simulink model "drone_nonlinear_full_compare"  (R2018a)
settings: Solver=VariableStepAuto  StartTime=0.0  StopTime=20  RelTol=1e-3
undefined symbols (not defined in the file): c, est_c_A, est_c_B, est_c_C, est_c_D, g, Ix, Iy, Iz, l, m, q, rpm, simulation_sampling_ts
libraries: simulink x8
settings Model: Creator=ros  LastModifiedBy=ros

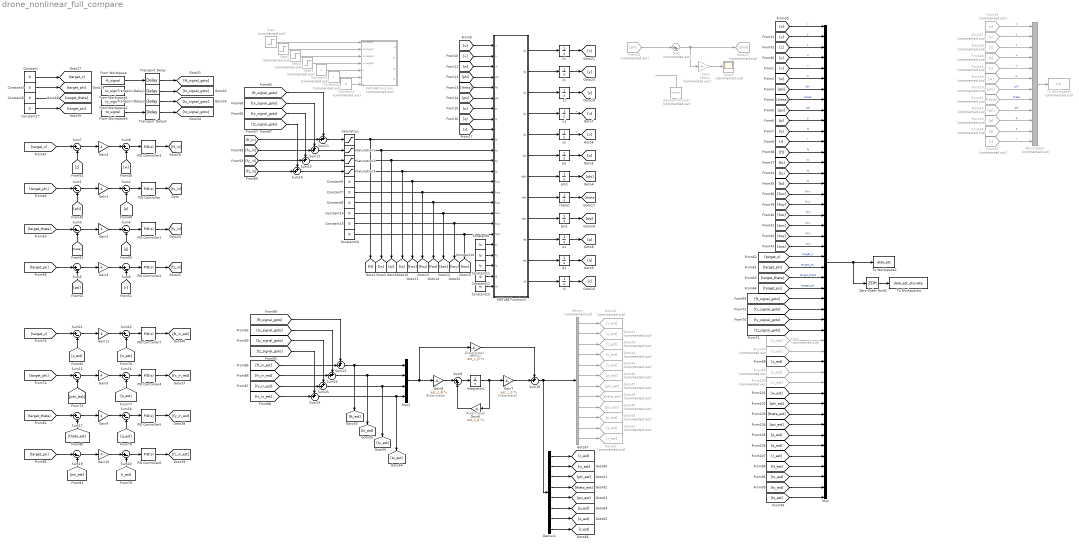
== system drone_nonlinear_full_compare ==
  note: B(estimate)
  note: C(estimate)
  note: A(estimate)
  note: D(estimate)
  Bus Creator : BusCreator  Commented=on  Inputs=12
  Constant{,3,5..8,14..17} (10 alike) : Constant  Value=0
  Constant1 : Constant  Commented=on  Value=l
  Constant10 : Constant  Value=Iy
  Constant11 : Constant  Value=Iz
  Constant12 : Constant  Value=g
  Constant13 : Constant  Value=m
  Constant2 : Constant  Commented=on  Value=c
  Constant4 : Constant  Commented=on  Value=q
  Constant9 : Constant  Value=Ix
  Demux : Demux  Commented=on  Outputs=12
  Demux1 : Demux  Outputs=8
  From : From  Commented=on  GotoTag=x_est
  From Workspace : FromWorkspace  VariableName=ft_signal  SampleTime=0
  From Workspace1 : FromWorkspace  VariableName=tx_signal  SampleTime=0
  From Workspace2 : FromWorkspace  VariableName=ty_signal  SampleTime=0
  From Workspace3 : FromWorkspace  VariableName=tz_signal  SampleTime=0
  From100 : From  Commented=on  GotoTag=v_est
  From18 : From  Commented=on  GotoTag=v
  From19 : From  Commented=on  GotoTag=w
  From20 : From  Commented=on  GotoTag=phi
  From21 : From  Commented=on  GotoTag=theta
  From22 : From  Commented=on  GotoTag=psi
  From23 : From  Commented=on  GotoTag=p
  From24 : From  Commented=on  GotoTag=q
  From25 : From  Commented=on  GotoTag=r
  From26 : From  Commented=on  GotoTag=u
  From27 : From  Commented=on  GotoTag=y
  From28 : From  Commented=on  GotoTag=z
  From29 : From  Commented=on  GotoTag=x
  From44 : From  Commented=on  GotoTag=phi
  From97 : From  Commented=on  GotoTag=y_est
  From99 : From  Commented=on  GotoTag=u_est
  Gain : Gain  Commented=on  Gain=180/pi
  Gain{1..5,9..11} (8 alike) : Gain  Gain=4
  Gain12 : Gain  Gain=est_c_D  Multiplication=Matrix(K*u)
  Gain6 : Gain  Gain=est_c_A  Multiplication=Matrix(K*u)
  Gain7 : Gain  Gain=est_c_C  Multiplication=Matrix(K*u)
  Gain8 : Gain  Gain=est_c_B  Multiplication=Matrix(K*u)
  Goto23 : Goto  Commented=on  GotoTag=phid
  Goto41 : Goto  Commented=on  GotoTag=x_est
  Goto42 : Goto  Commented=on  GotoTag=y_est
  Goto43 : Goto  Commented=on  GotoTag=z_est
  Goto44 : Goto  Commented=on  GotoTag=u_est
  Goto45 : Goto  Commented=on  GotoTag=v_est
  Goto46 : Goto  Commented=on  GotoTag=w_est
  Goto47 : Goto  Commented=on  GotoTag=phi_est
  Goto48 : Goto  Commented=on  GotoTag=theta_est
  Goto49 : Goto  Commented=on  GotoTag=psi_est
  Goto50 : Goto  Commented=on  GotoTag=p_est
  Goto51 : Goto  Commented=on  GotoTag=q_est
  Goto52 : Goto  Commented=on  GotoTag=r_est
  Integrator1 : Integrator
  MATLAB Function : MATLAB Function  Commented=on  TreatAsAtomicUnit=on
  MATLAB Function2 : MATLAB Function  TreatAsAtomicUnit=on
  Mux : Mux  Inputs=46
  Mux1 : Mux
  PID Controller{,1..2,4..6} (6 alike) : simulink/Continuous/PID Controller  Controller=PID  TimeDomain=Continuous-time  SampleTime=-1  IntegratorMethod=Forward Euler  FilterMethod=Forward Euler  Form=Parallel  UseFilter=on  ControllerParametersSource=internal  P=1.5  I=1.5  D=0  N=100  InitialConditionSource=internal  InitialConditionForIntegrator=0  InitialConditionForFilter=0  ExternalReset=none  LimitOutput=off  UpperSaturationLimit=inf  LowerSaturationLimit=-inf  LinearizeAsGain=on  AntiWindupMode=none  Kb=1  TrackingMode=off  Kt=1  PParamMin=[]  PParamMax=[]  IParamMin=[]  IParamMax=[]  DParamMin=[]  DParamMax=[]  NParamMin=[]  NParamMax=[]  KbParamMin=[]  KbParamMax=[]  KtParamMin=[]  KtParamMax=[]  POutMin=[]  POutMax=[]  IOutMin=[]  IOutMax=[]  DOutMin=[]  DOutMax=[]  NOutMin=[]  NOutMax=[]  KbOutMin=[]  KbOutMax=[]  KtOutMin=[]  KtOutMax=[]  IntegratorOutMin=[]  IntegratorOutMax=[]  FilterOutMin=[]  FilterOutMax=[]  SumOutMin=[]  SumOutMax=[]  SumI1OutMin=[]  SumI1OutMax=[]  SumI2OutMin=[]  SumI2OutMax=[]  SumI3OutMin=[]  SumI3OutMax=[]  SumDOutMin=[]  SumDOutMax=[]  SaturationOutMin=[]  SaturationOutMax=[]  IntegratorContinuousStateAttributes=''  IntegratorStateMustResolveToSignalObject=off  IntegratorRTWStateStorageClass=Auto  FilterContinuousStateAttributes=''  FilterStateMustResolveToSignalObject=off  FilterRTWStateStorageClass=Auto  DifferentiatorICPrevScaledInput=0  DifferentiatorOutMin=[]  DifferentiatorOutMax=[]  FilterDiffOutCoefMin=[]  FilterDiffOutCoefMax=[]  SumDenOutMin=[]  SumDenOutMax=[]  SumNumOutMin=[]  SumNumOutMax=[]  ReciprocalOutMin=[]  ReciprocalOutMax=[]  DivideOutMin=[]  DivideOutMax=[]  TunerSelectOption=Transfer Function Based (PID Tuner App)
  PID Controller3 : simulink/Continuous/PID Controller  Controller=PID  TimeDomain=Continuous-time  SampleTime=-1  IntegratorMethod=Forward Euler  FilterMethod=Forward Euler  Form=Parallel  UseFilter=on  ControllerParametersSource=internal  P=7  I=6  D=0.7  N=100  InitialConditionSource=internal  InitialConditionForIntegrator=0  InitialConditionForFilter=0  ExternalReset=none  LimitOutput=off  UpperSaturationLimit=inf  LowerSaturationLimit=-inf  LinearizeAsGain=on  AntiWindupMode=none  Kb=1  TrackingMode=off  Kt=1  PParamMin=[]  PParamMax=[]  IParamMin=[]  IParamMax=[]  DParamMin=[]  DParamMax=[]  NParamMin=[]  NParamMax=[]  KbParamMin=[]  KbParamMax=[]  KtParamMin=[]  KtParamMax=[]  POutMin=[]  POutMax=[]  IOutMin=[]  IOutMax=[]  DOutMin=[]  DOutMax=[]  NOutMin=[]  NOutMax=[]  KbOutMin=[]  KbOutMax=[]  KtOutMin=[]  KtOutMax=[]  IntegratorOutMin=[]  IntegratorOutMax=[]  FilterOutMin=[]  FilterOutMax=[]  SumOutMin=[]  SumOutMax=[]  SumI1OutMin=[]  SumI1OutMax=[]  SumI2OutMin=[]  SumI2OutMax=[]  SumI3OutMin=[]  SumI3OutMax=[]  SumDOutMin=[]  SumDOutMax=[]  SaturationOutMin=[]  SaturationOutMax=[]  IntegratorContinuousStateAttributes=''  IntegratorStateMustResolveToSignalObject=off  IntegratorRTWStateStorageClass=Auto  FilterContinuousStateAttributes=''  FilterStateMustResolveToSignalObject=off  FilterRTWStateStorageClass=Auto  DifferentiatorICPrevScaledInput=0  DifferentiatorOutMin=[]  DifferentiatorOutMax=[]  FilterDiffOutCoefMin=[]  FilterDiffOutCoefMax=[]  SumDenOutMin=[]  SumDenOutMax=[]  SumNumOutMin=[]  SumNumOutMax=[]  ReciprocalOutMin=[]  ReciprocalOutMax=[]  DivideOutMin=[]  DivideOutMax=[]  TunerSelectOption=Transfer Function Based (PID Tuner App)
  PID Controller7 : simulink/Continuous/PID Controller  Controller=PID  TimeDomain=Continuous-time  SampleTime=-1  IntegratorMethod=Forward Euler  FilterMethod=Forward Euler  Form=Parallel  UseFilter=on  ControllerParametersSource=internal  P=7  I=6  D=0.7  N=100  InitialConditionSource=internal  InitialConditionForIntegrator=0  InitialConditionForFilter=0  ExternalReset=none  LimitOutput=off  UpperSaturationLimit=inf  LowerSaturationLimit=-inf  LinearizeAsGain=on  AntiWindupMode=none  Kb=1  TrackingMode=off  Kt=1  PParamMin=[]  PParamMax=[]  IParamMin=[]  IParamMax=[]  DParamMin=[]  DParamMax=[]  NParamMin=[]  NParamMax=[]  KbParamMin=[]  KbParamMax=[]  KtParamMin=[]  KtParamMax=[]  POutMin=[]  POutMax=[]  IOutMin=[]  IOutMax=[]  DOutMin=[]  DOutMax=[]  NOutMin=[]  NOutMax=[]  KbOutMin=[]  KbOutMax=[]  KtOutMin=[]  KtOutMax=[]  IntegratorOutMin=[]  IntegratorOutMax=[]  FilterOutMin=[]  FilterOutMax=[]  SumOutMin=[]  SumOutMax=[]  SumI1OutMin=[]  SumI1OutMax=[]  SumI2OutMin=[]  SumI2OutMax=[]  SumI3OutMin=[]  SumI3OutMax=[]  SumDOutMin=[]  SumDOutMax=[]  SaturationOutMin=[]  SaturationOutMax=[]  IntegratorContinuousStateAttributes=''  IntegratorStateMustResolveToSignalObject=off  IntegratorRTWStateStorageClass=Auto  FilterContinuousStateAttributes=''  FilterStateMustResolveToSignalObject=off  FilterRTWStateStorageClass=Auto  DifferentiatorICPrevScaledInput=0  DifferentiatorOutMin=[]  DifferentiatorOutMax=[]  FilterDiffOutCoefMin=[]  FilterDiffOutCoefMax=[]  SumDenOutMin=[]  SumDenOutMax=[]  SumNumOutMin=[]  SumNumOutMax=[]  ReciprocalOutMin=[]  ReciprocalOutMax=[]  DivideOutMin=[]  DivideOutMax=[]  TunerSelectOption=Transfer Function Based (PID Tuner App)
  Random Number : RandomNumber  Commented=on  Variance=0.00001
  Saturation{,1..3} (4 alike) : Saturate  UpperLimit=30  LowerLimit=-100
  Scope : Scope  Commented=on
  Step{,1..3} (4 alike) : Step  Commented=on  Time=0  After=rpm  SampleTime=0
  Sum : Sum  Commented=on  Inputs=|++
  Sum{1..8,15..22} (16 alike) : Sum  Inputs=|+-
  Sum{10..14,23..26} (9 alike) : Sum  Inputs=++|
  Sum9 : Sum  Inputs=|++
  To Workspace1 : ToWorkspace  Commented=on  VariableName=out  SaveFormat=Timeseries  SampleTime=-1
  To Workspace2 : ToWorkspace  VariableName=data_est  SaveFormat=Timeseries  SampleTime=-1
  To Workspace4 : ToWorkspace  VariableName=data_est_discrete  SaveFormat=Timeseries  SampleTime=-1
  Transport Delay{,1..3} (4 alike) : TransportDelay  DelayTime=10
  Zero-Order Hold1 : ZeroOrderHold  SampleTime=simulation_sampling_ts
  p1 : Integrator
  phi1 : Integrator
  psi1 : Integrator
  q1 : Integrator
  r1 : Integrator
  theta1 : Integrator
  u1 : Integrator
  v1 : Integrator
  w1 : Integrator
  x1 : Integrator
  y1 : Integrator
  z1 : Integrator
  wires:
  [v] -> MATLAB Function2/2(v)
  MATLAB Function2/9(dps) -> psi1/1
  MATLAB Function2/10(dp) -> p1/1
  MATLAB Function2/5(dv) -> v1/1
  [r] -> MATLAB Function2/9(r)
  [psi] -> MATLAB Function2/6(ps)
  [ft_in] -> Sum11/2
  [p] -> MATLAB Function2/7(p)
  p1/1 -> [p]
  MATLAB Function2/12(dr) -> r1/1
  theta1/1 -> [theta]
  [w] -> MATLAB Function2/3(w)
  [phi] -> MATLAB Function2/4(ph)
  [q] -> MATLAB Function2/8(q)
  r1/1 -> [r]
  q1/1 -> [q]
  MATLAB Function2/11(dq) -> q1/1
  MATLAB Function2/6(dw) -> w1/1
  MATLAB Function2/4(du) -> u1/1
  psi1/1 -> [psi]
  [u] -> MATLAB Function2/1(u)
  MATLAB Function2/8(dth) -> theta1/1
  [theta] -> MATLAB Function2/5(th)
  u1/1 -> [u]  "u"
  w1/1 -> [w]
  MATLAB Function2/7(dph) -> phi1/1
  v1/1 -> [v]  "v"
  Constant9/1 -> MATLAB Function2/20(Ix)
  Constant13/1 -> MATLAB Function2/24(m)
  Constant11/1 -> MATLAB Function2/22(Iz)
  Constant10/1 -> MATLAB Function2/21(Iy)
  Constant12/1 -> MATLAB Function2/23(g)
  MATLAB Function2/1(dx) -> x1/1
  MATLAB Function2/2(dy) -> y1/1
  MATLAB Function2/3(dz) -> z1/1
  Constant6/1 -> [fwx], MATLAB Function2/14(fwx)
  Constant7/1 -> [fwy], MATLAB Function2/15(fwy)
  Constant14/1 -> [twx], MATLAB Function2/17(twx)
  Constant8/1 -> [fwz], MATLAB Function2/16(fwz)
  Constant15/1 -> [twy], MATLAB Function2/18(twy)
  Constant16/1 -> [twz], MATLAB Function2/19(twz)
  Bus Creator/1 -> To Workspace1/1
  z1/1 -> [z]
  y1/1 -> [y]
  x1/1 -> [x]
  From29/1 -> Bus Creator/1  "x"
  From27/1 -> Bus Creator/2  "y"
  From28/1 -> Bus Creator/3  "z"
  From26/1 -> Bus Creator/4  "u"
  From18/1 -> Bus Creator/5  "v"
  From19/1 -> Bus Creator/6  "w"
  From20/1 -> Bus Creator/7  "phi"
  From21/1 -> Bus Creator/8  "theta"
  From22/1 -> Bus Creator/9  "psi"
  From23/1 -> Bus Creator/10  "p"
  From24/1 -> Bus Creator/11  "q"
  From25/1 -> Bus Creator/12  "r"
  [x] -> Mux/1  "x"
  [v] -> Mux/5  "v"
  [z] -> Mux/3  "z"
  [w] -> Mux/6  "w"
  [p] -> Mux/10  "p"
  [phi] -> Mux/7  "phi"
  [theta] -> Mux/8  "theta"
  [r] -> Mux/12  "r"
  [y] -> Mux/2  "y"
  [psi] -> Mux/9  "psi"
  [u] -> Mux/4  "u"
  [q] -> Mux/11  "q"
  Mux/1 -> Zero-Order Hold1/1, To Workspace2/1
  [ft] -> Mux/13  "ft"
  [tx] -> Mux/14  "tx"
  [ty] -> Mux/15  "ty"
  [tz] -> Mux/16  "tz"
  [fwx] -> Mux/17  "fwx"
  [fwy] -> Mux/18  "fwy"
  [fwz] -> Mux/19  "fwz"
  [twx] -> Mux/20  "twx"
  [twy] -> Mux/21  "twy"
  [twz] -> Mux/22  "twz"
  phi1/1 -> [phi]
  Random Number/1 -> ?
  From44/1 -> Sum/1
  Gain/1 -> Scope/1
  Sum/1 -> Goto23/1, Gain/1
  Zero-Order Hold1/1 -> To Workspace4/1
  Constant1/1 -> MATLAB Function/6(l)
  Constant2/1 -> MATLAB Function/5(c)
  Constant4/1 -> MATLAB Function/7(q)
  Step/1 -> MATLAB Function/1(omega1)
  Step1/1 -> MATLAB Function/2(omega2)
  Step2/1 -> MATLAB Function/3(omega3)
  Step3/1 -> MATLAB Function/4(omega4)
  [phi] -> Sum1/2
  [target_phi] -> Sum1/1
  Sum1/1 -> Gain1/1
  Gain1/1 -> Sum2/1
  Sum2/1 -> PID Controller/1
  [p] -> Sum2/2
  [q] -> Sum4/2
  Gain2/1 -> Sum4/1
  [target_theta] -> Sum3/1
  Sum4/1 -> PID Controller1/1
  Sum3/1 -> Gain2/1
  [theta] -> Sum3/2
  [r] -> Sum6/2
  Gain3/1 -> Sum6/1
  [target_psi] -> Sum5/1
  Sum6/1 -> PID Controller2/1
  Sum5/1 -> Gain3/1
  [psi] -> Sum5/2
  [target_z] -> Sum7/1
  Sum8/1 -> PID Controller3/1
  [w] -> Sum8/2
  Sum7/1 -> Gain4/1
  Gain4/1 -> Sum8/1
  [z] -> Sum7/2
  PID Controller/1 -> [fx_in]
  PID Controller2/1 -> [fz_in]
  PID Controller1/1 -> [fy_in]
  PID Controller3/1 -> [ft_in]
  Saturation/1 -> [ft], MATLAB Function2/10(ft)
  Saturation1/1 -> [tx], MATLAB Function2/11(tx)
  Saturation2/1 -> [ty], MATLAB Function2/12(ty)
  Saturation3/1 -> [tz], MATLAB Function2/13(tz)
  [target_z] -> Mux/23  "target_z"
  [target_phi] -> Mux/24  "target_phi"
  [target_theta] -> Mux/25  "target_theta"
  [target_psi] -> Mux/26  "target_psi"
  Sum11/1 -> Saturation/1
  [fx_in] -> Sum12/2
  Sum12/1 -> Saturation1/1
  Sum13/1 -> Saturation2/1
  [fy_in] -> Sum13/2
  Sum14/1 -> Saturation3/1
  [fz_in] -> Sum14/2
  [ft_signal_goto] -> Sum11/1
  [tx_signal_goto] -> Sum12/1
  [ty_signal_goto] -> Sum13/1
  [tz_signal_goto] -> Sum14/1
  Constant17/1 -> [target_psi]
  Constant5/1 -> [target_theta]
  Constant/1 -> [target_z]
  Constant3/1 -> [target_phi]
  [tx_signal_goto] -> Mux/28
  [ty_signal_goto] -> Mux/29
  [tz_signal_goto] -> Mux/30
  [ft_signal_goto] -> Mux/27
  Mux1/1 -> Gain12/1, Gain8/1
  Sum9/1 -> Integrator1/1
  Integrator1/1 -> Gain7/1, Gain6/1
  Gain8/1 -> Sum9/1
  Gain6/1 -> Sum9/2
  Gain7/1 -> Sum10/2
  [q_est] -> Sum18/2
  PID Controller6/1 -> [fz_in_est]
  [target_phi] -> Sum15/1
  PID Controller7/1 -> [ft_in_est]
  PID Controller5/1 -> [fy_in_est]
  Gain5/1 -> Sum16/1
  [target_psi] -> Sum19/1
  Sum20/1 -> PID Controller6/1
  Sum22/1 -> PID Controller7/1
  [p_est] -> Sum16/2
  Sum21/1 -> Gain11/1
  [w_est] -> Sum22/2
  [z_est] -> Sum21/2
  PID Controller4/1 -> [fx_in_est]
  [phi_est] -> Sum15/2
  Sum17/1 -> Gain9/1
  Sum18/1 -> PID Controller5/1
  [target_theta] -> Sum17/1
  [theta_est] -> Sum17/2
  [r_est] -> Sum20/2
  [psi_est] -> Sum19/2
  [target_z] -> Sum21/1
  Gain10/1 -> Sum20/1
  Sum15/1 -> Gain5/1
  Sum19/1 -> Gain10/1
  Gain9/1 -> Sum18/1
  Gain11/1 -> Sum22/1
  Sum16/1 -> PID Controller4/1
  [tz_signal_goto] -> Sum26/1
  [ty_signal_goto] -> Sum25/1
  [tx_signal_goto] -> Sum24/1
  [ft_signal_goto] -> Sum23/1
  Sum26/1 -> [tz_est], Mux1/4
  [fz_in_est] -> Sum26/2
  Sum24/1 -> Mux1/2, [tx_est]
  [ft_in_est] -> Sum23/2
  [fy_in_est] -> Sum25/2
  [fx_in_est] -> Sum24/2
  Sum23/1 -> Mux1/1, [ft_est]
  Sum25/1 -> Mux1/3, [ty_est]
  Demux/1 -> Goto41/1
  Demux/2 -> Goto42/1
  Demux/3 -> Goto43/1
  Demux/4 -> Goto44/1
  Demux/5 -> Goto45/1
  Demux/6 -> Goto46/1
  Demux/7 -> Goto47/1
  Demux/8 -> Goto48/1
  Demux/9 -> Goto49/1
  Demux/10 -> Goto50/1
  Demux/11 -> Goto51/1
  Demux/12 -> Goto52/1
  [ty_est] -> Mux/45
  [ft_est] -> Mux/43
  [tx_est] -> Mux/44
  [tz_est] -> Mux/46
  From/1 -> Mux/31
  From97/1 -> Mux/32
  [z_est] -> Mux/33
  From99/1 -> Mux/34
  From100/1 -> Mux/35
  [w_est] -> Mux/36
  [phi_est] -> Mux/37
  [theta_est] -> Mux/38
  [psi_est] -> Mux/39
  [p_est] -> Mux/40
  [q_est] -> Mux/41
  [r_est] -> Mux/42
  Gain12/1 -> Sum10/1
  From Workspace/1 -> Transport Delay/1
  From Workspace1/1 -> Transport Delay1/1
  From Workspace2/1 -> Transport Delay2/1
  From Workspace3/1 -> Transport Delay3/1
  Transport Delay/1 -> [ft_signal_goto]
  Transport Delay1/1 -> [tx_signal_goto]
  Transport Delay2/1 -> [ty_signal_goto]
  Transport Delay3/1 -> [tz_signal_goto]
  Sum10/1 -> Demux1/1, Demux/1
  Demux1/1 -> [z_est]
  Demux1/2 -> [w_est]
  Demux1/3 -> [phi_est]
  Demux1/4 -> [theta_est]
  Demux1/5 -> [psi_est]
  Demux1/6 -> [p_est]
  Demux1/7 -> [q_est]
  Demux1/8 -> [r_est]

== matlab function drone_nonlinear_full_compare/MATLAB Function ==
  data: omega1 input; ft output; omega2 input; omega3 input; omega4 input; c input; l input; q input; tx output; ty output; tz output
function [ft,tx,ty,tz] = fcn(omega1,omega2,omega3,omega4,c,l,q)
ft = c*(omega1^2 + omega2^2 + omega3^2 + omega4^2);
tx = c*l*(omega1^2 - omega2^2 - omega3^2 + omega4^2);
ty = c*l*(omega1^2 + omega2^2 - omega3^2 - omega4^2);
tz = q*(-omega1^2 + omega2^2 - omega3^2 + omega4^2);

== matlab function drone_nonlinear_full_compare/MATLAB Function2 ==
  data: u input; v input; dx output; w input; ph input; th input; ps input; p input; q input; r input; ft input; tx input; ty input; tz input; fwx input; fwy input; fwz input; twx input; twy input; twz input; dy output; dz output; du output; dv output; dw output; dph output; dth output; dps output; dp output; dq output; dr output; Ix input; Iy input; Iz input; g input; m input
function [dx, dy, dz, du, dv, dw, dph, dth, dps, dp, dq, dr] = fcn(u, v, w, ph, th, ps, p, q, r, ft, tx, ty, tz, fwx, fwy, fwz, twx, twy, twz, Ix, Iy, Iz, g, m)

dx = w*(sin(ph)*sin(ps) + cos(ph)*cos(ps)*sin(th)) - v*(cos(ph)*sin(ps) - cos(ps)*sin(ph)*sin(th)) + u*(cos(ps)*cos(th));
dy = v*(cos(ph)*cos(ps) + sin(ph)*sin(ps)*sin(th)) - w*(cos(ps)*sin(ph) - cos(ph)*sin(ps)*sin(th)) + u*(cos(th)*sin(ps));
dz = w*(cos(ph)*cos(th)) - u*(sin(th)) + v*(cos(th)*sin(ph));
du = r*v - q*w + g*(sin(th)) + fwx / m;
dv = p*w - r*u - g*(sin(ph)*cos(th)) + fwy / m;
dw = q*u - p*v - g*(cos(th)*cos(ph)) + (fwz + ft) / m;
dph = p + r*(cos(ph)*tan(th)) + q*(sin(ph)*tan(th));
dth = q*(cos(th)) - r*(sin(ph));
dps = r*(cos(ph)/cos(th)) + q*(sin(ph)/cos(th));
dp = r*q*(Iy - Iz)/Ix + (tx + twx)/Ix;
dq = p*r*(Iz - Ix)/Iy + (ty + twy)/Iy;
dr = p*q*(Ix - Iy)/Iz + (tz + twz)/Iz;
